simulink model "SGBMDisparity"  (R2021a)
settings: Solver=FixedStepDiscrete  StartTime=0.0  StopTime=simT  FixedStep=1  RelTol=1e-3
PreLoadFcn:
  | DL128 = Simulink.Variant('disparityLevels==128');
  | 
  | DLnot128 = Simulink.Variant('disparityLevels ~= 128');
  | 
  | disparityLevels = 64;
  | 
  | imgRowSize = 480;
  | 
  | imgColSize = 640;
  | 
  | P2 = 200; % Smoothness Penalty Large
  | P1 = 15;  % Smoothness Penalty Small
  | 
  | disparityFactor = 16;
  | 
  | uniquenessRatio = 5;
  | 
  | p = imgColSize - 1;
  | q = imgRowSize * imgColSize -1;
  | r = imgColSize - disparityLevels -1;
  | s = (imgRowSize*(imgColSize-disparityLevels))-1;
  | 
  | simT = 800*525
  | 
  | dtGain = 4;
InitFcn:
  | DL128 = Simulink.Variant('disparityLevels==128');
  | 
  | DLnot128 = Simulink.Variant('disparityLevels ~= 128');
  | 
  | img = imread(get_param('SGBMDisparity/stereoImage','FileName'));
  | 
  | [imgRowSize, imgColSize,chn] = size(img);
  | 
  | P2 = 200; % Smoothness Penalty Large
  | P1 = 15;  % Smoothness Penalty Small
  | 
  | disparityFactor = 16;
  | 
  | uniquenessRatio = str2num(get_param('SGBMDisparity/SGBMHDLAlgorithm/SGBMHDLAlgorithmWorker','UT'));
  | 
  | disparityLevels = str2num(get_param('SGBMDisparity/SGBMHDLAlgorithm/SGBMHDLAlgorithmWorker','DL'));
  | 
  | p = imgColSize - 1;
  | q = imgRowSize * imgColSize -1;
  | r = imgColSize - disparityLevels -1;
  | s = (imgRowSize*(imgColSize-disparityLevels))-1;
  | 
  | if imgRowSize == 720 && imgColSize == 1280
  | simT = 1650*750;
  | elseif imgRowSize == 540 && imgColSize == 960
  | simT = 1050*600;
  | elseif imgRowSize == 480 && imgColSize == 640
  | simT = 800*525;
  | end
  | 
  | %if imgRowSize == 720 && imgColSize == 1280
  | %dtGain = 2;
  | %elseif imgRowSize == 540 && imgColSize == 960
  | %dtGain = 2.6;
  | %elseif imgRowSize == 480 && imgColSize == 640
  | %dtGain = 4;
  | %end
  | 
  | dtGain = 8;
libraries: simulink x331, hdlsllib x113, visionhdlutilities x9, visionhdlio x2, visionsources x1
(part 1 of 6)
settings Model: DataTypeOverride=Off  SimulationMode=accelerator  Creator=The MathWorks, Inc.  LastModifiedBy=user
settings SolverCC: AlgebraicLoopSolver=TrustRegion  AutoInsertRateTranBlk=on
settings DataIOCC: LimitDataPoints=on  SaveOutput=off  SignalLogging=off  SaveTime=off  ReturnWorkspaceOutputs=off
settings OptimizationCC: BlockReduction=off  ConditionallyExecuteInputs=off  DefaultParameterBehavior=Inlined  LifeSpan=inf
settings DebuggingCC: AlgebraicLoopMsg=error  SingleTaskRateTransMsg=error  AllowSymbolicDim=off  StrictBusMsg=ErrorOnBusTreatedAsVector  SFUnexpectedBacktrackingDiag=warning  SFNoUnconditionalDefaultTransitionDiag=warning  SFExecutionAtInitializationDiag=none  SFMachineParentedDataDiag=warning  ArithmeticOperatorsInVariantConditions=warning
settings HardwareCC: ProdBitPerPointer=32  ProdBitPerSizeT=32  ProdBitPerPtrDiffT=32  ProdLargestAtomicFloat=None  ProdIntDivRoundTo=Undefined  ProdEndianess=Unspecified  ProdWordSize=32  ProdHWDeviceType=ASIC/FPGA->ASIC/FPGA  ProdEqTarget=off
settings SFSimCC: SimUseLocalCustomCode=off  CustomCodeUndefinedFunction=UseInterfaceOnly
settings RTWCC: RTWUseLocalCustomCode=off
settings CodeAppCC: StateflowObjectComments=on
settings GRTTargetCC: TargetLangStandard=C89/C90 (ANSI)
settings ConfigComp: CovMetricSettings=dw  CovSaveCumulativeToWorkspaceVar=on  CovSaveSingleToWorkspaceVar=on  CovExternalEMLEnable=off  CovSFcnEnable=off

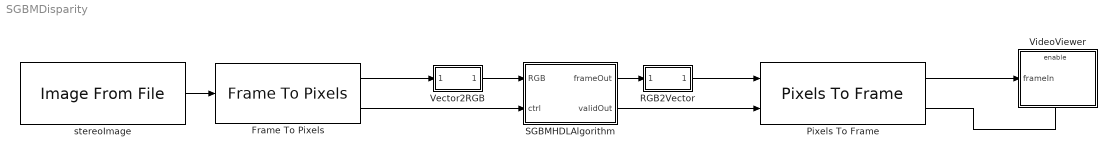
== system SGBMDisparity ==
  Frame To Pixels : visionhdlio/Frame To Pixels  NumComponents=3  NumPixels=1  VideoFormat=480p  ActivePixelsPerLine=imgColSize  ActiveVideoLines=imgRowSize  TotalPixelsPerLine=imgColSize+90  TotalVideoLines=imgRowSize+60  StartingActiveLine=31  FrontPorch=45  SampleTime=0
      settings: SourceProductBaseCode=VT
  Pixels To Frame : visionhdlio/Pixels To Frame  NumComponents=3  NumPixels=1  VideoFormat=480p  ActivePixelsPerLine=imgColSize  ActiveVideoLines=imgRowSize  TotalPixelsPerLine=imgColSize+90  TotalVideoLines=imgRowSize+60
      settings: SourceProductBaseCode=VT
  RGB2Vector : Subsystem
  SGBMHDLAlgorithm : Subsystem  TreatAsAtomicUnit=on
  Vector2RGB : Subsystem
  VideoViewer : Subsystem
  stereoImage : visionsources/Image From File  Tag=vipblks_nd  FileName=D:\Work\XilFPGAdev\Custom_IP_Cores\SimulinkHDLCoder\SGBMDisparity\stereoTestimg_01_480p.bmp  Ts=simT  imagePorts=One multidimensional signal  OutPortLabels=R|G|B  ImageDataType=Inherit from input image  sdImageDataType=uint(8)  Signed=on  WordLength=16  FractionLengthMode=User-defined  FractionLength=15
  wires:
  stereoImage/1 -> Frame To Pixels/1
  Pixels To Frame/1 -> VideoViewer/1(frameIn)
  Pixels To Frame/2 -> VideoViewer/Enable
  Frame To Pixels/1 -> Vector2RGB/1(RGBVector)
  Frame To Pixels/2 -> SGBMHDLAlgorithm/2(ctrl)
  SGBMHDLAlgorithm/1(frameOut) -> RGB2Vector/1(RGB)
  SGBMHDLAlgorithm/2(validOut) -> Pixels To Frame/2
  Vector2RGB/1(RGB) -> SGBMHDLAlgorithm/1(RGB)
  RGB2Vector/1(RGBVector) -> Pixels To Frame/1

== system SGBMDisparity/RGB2Vector ==
  note: RGB represented in
      | 32'hFFRRGGBB
  RGB : Inport
  Bit Slice : hdlsllib/Logic and Bit Operations/Bit Slice  lidx=23  ridx=16
      settings: SourceProductBaseCode=SL
  Bit Slice1 : hdlsllib/Logic and Bit Operations/Bit Slice  lidx=15  ridx=8
      settings: SourceProductBaseCode=SL
  Bit Slice2 : hdlsllib/Logic and Bit Operations/Bit Slice  lidx=7  ridx=0
      settings: SourceProductBaseCode=SL
  Mux : Mux  Inputs=3
  Signal Specification : SignalSpecification
  Transpose : Math  Operator=transpose  SignedPower=on  SaturateOnIntegerOverflow=on
  RGBVector : Outport  VectorParamsAs1DForOutWhenUnconnected=off
  wires:
  Mux/1 -> Transpose/1
  Bit Slice/1 -> Mux/1
  Bit Slice2/1 -> Mux/3
  Bit Slice1/1 -> Mux/2
  RGB/1 -> Bit Slice2/1, Bit Slice1/1, Bit Slice/1
  Transpose/1 -> Signal Specification/1
  Signal Specification/1 -> RGBVector/1

== system SGBMDisparity/SGBMHDLAlgorithm ==
  RGB : Inport
  ctrl : Inport  Port=2
  Bit Concat : hdlsllib/Logic and Bit Operations/Bit Concat  numInputs=4
  Demux : Demux  Outputs=3
  FF : Constant  Value=255  OutDataTypeStr=uint8  SampleTime=-1
  Output : Subsystem
  RGB2Vector : Subsystem
  SGBMHDLAlgorithmWorker : Subsystem  mask{DL=16, UT=5}
      mask prompts: DL "Disparity Levels"; UT "Uniqueness Threshold"
      mask DialogControl Container3 Prompt: Select Disparity Levels
      mask DialogControl Container6 Prompt: Select Uniqueness Threshold
  frameOut : Outport
  validOut : Outport  Port=2
  wires:
  Output/2(validOut) -> validOut/1
  Demux/2 -> SGBMHDLAlgorithmWorker/2(pixelRight)
  SGBMHDLAlgorithmWorker/2(ctrlDisparity) -> Output/2(busIn)
  Demux/1 -> SGBMHDLAlgorithmWorker/1(pixelLeft)
  SGBMHDLAlgorithmWorker/1(pixelDisparity) -> Output/1(pixelIn)
  ctrl/1 -> SGBMHDLAlgorithmWorker/3(ctrl)
  RGB/1 -> RGB2Vector/1(RGB)
  RGB2Vector/1(RGBVector) -> Demux/1
  Bit Concat/1 -> frameOut/1
  FF/1 -> Bit Concat/1
  Output/1(frameOut) -> Bit Concat/4, Bit Concat/2, Bit Concat/3

== system SGBMDisparity/Vector2RGB ==
  note: Encode RGB into 32 bit representation
      | 32'hFFRRGGBB
  RGBVector : Inport
  Bit Concat : hdlsllib/Logic and Bit Operations/Bit Concat  numInputs=4
  Demux : Demux  Outputs=3
  FF : Constant  Value=255  OutDataTypeStr=uint8  SampleTime=-1
  RGB : Outport  VectorParamsAs1DForOutWhenUnconnected=off
  wires:
  Bit Concat/1 -> RGB/1
  RGBVector/1 -> Demux/1
  FF/1 -> Bit Concat/1
  Demux/1 -> Bit Concat/2
  Demux/2 -> Bit Concat/3
  Demux/3 -> Bit Concat/4

== system SGBMDisparity/VideoViewer ==
  frameIn : Inport
  Enable : EnablePort
  HDL Video Viewer : VideoViewer  useColorMap=on  FigPos=[348 749 756 478]
  wires:
  frameIn/1 -> HDL Video Viewer/1

== system SGBMDisparity/SGBMHDLAlgorithm/Output ==
  pixelIn : Inport
  busIn : Inport  Port=2
  Bus Selector : BusSelector  OutputSignals=valid,vStart
  Compare To Constant : simulink/Logic and Bit Operations/Compare To Constant  relop=<=  const=imgColSize-1  OutDataTypeStr=boolean
  Compare To Constant1 : simulink/Logic and Bit Operations/Compare To Constant  relop=<=  const=disparityLevels-1  OutDataTypeStr=boolean
  Constant : Constant  Value=0  OutDataTypeStr=boolean  SampleTime=-1
  Constant1 : Constant  OutDataTypeStr=boolean  SampleTime=-1
  Constant2 : Constant  Value=0  OutDataTypeStr=fixdt(1,14,5)  SampleTime=-1
  Data Type Conversion : DataTypeConversion  OutDataTypeStr=uint8
  Gain : Gain  Gain=dtGain
  HDL Counter : hdlsllib/Sources/HDL Counter  CountType=Count limited  CountInit=0  CountStep=1  CountMax=imgColSize-1  CountFromType=Initial value  CountFrom=0  CountResetPort=off  CountLoadPort=off  CountEnbPort=on  CountDirPort=off  CountHitOutputPort=off  CountDataType=Unsigned  CountWordLen=ceil(log2(imgColSize-1))  CountFracLen=0  CountSampTime=1
  Logical Operator : Logic  AllPortsSameDT=off  OutDataTypeStr=boolean
  Logical Operator1 : Logic  Operator=OR  AllPortsSameDT=off  OutDataTypeStr=boolean
  Logical Operator2 : Logic  Operator=OR  AllPortsSameDT=off  OutDataTypeStr=boolean
  Switch : Switch  Criteria=u2 ~= 0
  Switch1 : Switch  Criteria=u2 ~= 0
  Terminator : Terminator
  To Workspace : ToWorkspace  VariableName=dispMap  SampleTime=-1
      settings: Save2DSignal=2-D array (concatenate along first dimension)
  To Workspace1 : ToWorkspace  VariableName=dispMapValid  SampleTime=-1
      settings: Save2DSignal=2-D array (concatenate along first dimension)
  pixelBusGenerator : Subsystem  mask{hEnd=p, vEnd=q}
      mask prompts: hEnd "hEnd Count"; vEnd "vEnd Count"
      mask DialogControl DescGroupVar Prompt: Counter Values
  frameOut : Outport  VectorParamsAs1DForOutWhenUnconnected=off
  validOut : Outport  Port=2  VectorParamsAs1DForOutWhenUnconnected=off
  wires:
  pixelBusGenerator/1(busOut) -> validOut/1
  Switch1/1 -> Gain/1, To Workspace/1
  busIn/1 -> Bus Selector/1
  Gain/1 -> Data Type Conversion/1
  Data Type Conversion/1 -> frameOut/1
  Constant/1 -> Switch/3
  Constant1/1 -> Switch/1
  HDL Counter/1 -> Compare To Constant/1, Compare To Constant1/1
  Compare To Constant/1 -> Logical Operator/2
  Logical Operator1/1 -> HDL Counter/1
  Compare To Constant1/1 -> Logical Operator2/2, Logical Operator1/2
  Bus Selector/1 -> Switch1/2, Logical Operator/1, Logical Operator1/1  "<valid>"
  Logical Operator/1 -> Logical Operator2/1
  Logical Operator2/1 -> Switch/2
  Constant2/1 -> Switch1/3
  pixelIn/1 -> Switch1/1
  Switch/1 -> To Workspace1/1, pixelBusGenerator/1(validIn)
  Bus Selector/2 -> Terminator/1  "<vStart>"

== system SGBMDisparity/SGBMHDLAlgorithm/RGB2Vector ==
  note: RGB represented in
      | 32'hFFRRGGBB
  RGB : Inport
  Bit Slice : hdlsllib/Logic and Bit Operations/Bit Slice  lidx=23  ridx=16
      settings: SourceProductBaseCode=SL
  Bit Slice1 : hdlsllib/Logic and Bit Operations/Bit Slice  lidx=15  ridx=8
      settings: SourceProductBaseCode=SL
  Bit Slice2 : hdlsllib/Logic and Bit Operations/Bit Slice  lidx=7  ridx=0
      settings: SourceProductBaseCode=SL
  Mux : Mux  Inputs=3
  RGBVector : Outport  VectorParamsAs1DForOutWhenUnconnected=off
  wires:
  Bit Slice/1 -> Mux/1
  Bit Slice2/1 -> Mux/3
  Bit Slice1/1 -> Mux/2
  RGB/1 -> Bit Slice2/1, Bit Slice1/1, Bit Slice/1
  Mux/1 -> RGBVector/1

== system SGBMDisparity/SGBMHDLAlgorithm/SGBMHDLAlgorithmWorker ==
  pixelLeft : Inport
  pixelRight : Inport  Port=2
  ctrl : Inport  Port=3
  DirectionalCost : Subsystem
  MatchingCost : Subsystem
  PostProcessing : Subsystem
  pixelDisparity : Outport  VectorParamsAs1DForOutWhenUnconnected=off
  ctrlDisparity : Outport  Port=2  VectorParamsAs1DForOutWhenUnconnected=off
  wires:
  PostProcessing/1(disparityOut) -> pixelDisparity/1
  PostProcessing/2(busOut) -> ctrlDisparity/1
  pixelLeft/1 -> MatchingCost/1(pixelLeft)
  pixelRight/1 -> MatchingCost/2(pixelRight)
  ctrl/1 -> MatchingCost/3(busIn)
  MatchingCost/1(hammDistA) -> DirectionalCost/1(matchCostA)
  MatchingCost/2(hammDistValidA) -> DirectionalCost/2(busA)
  MatchingCost/3(hammDistRL) -> DirectionalCost/3(matchCostRL)
  MatchingCost/4(hammDistValidRL) -> DirectionalCost/4(busRL)
  DirectionalCost/2(validOut) -> PostProcessing/2(validIn)
  DirectionalCost/1(totalCostOut) -> PostProcessing/1(totalCostIn)

== system SGBMDisparity/SGBMHDLAlgorithm/Output/pixelBusGenerator ==
  validIn : Inport
  Horizontal : hdlsllib/Sources/HDL Counter  CountType=Count limited  CountInit=0  CountStep=1  CountMax=hEnd  CountFromType=Initial value  CountFrom=0  CountResetPort=off  CountLoadPort=off  CountEnbPort=on  CountDirPort=off  CountHitOutputPort=off  CountDataType=Unsigned  CountWordLen=ceil(log2(hEnd))  CountFracLen=0  CountSampTime=1
  Logical Operator{3..6} (4 alike) : Logic  AllPortsSameDT=off  OutDataTypeStr=boolean
  Pixel Control Bus Creator : visionhdlutilities/Pixel Control Bus Creator
      settings: SourceProductBaseCode=VT
  Vertical : hdlsllib/Sources/HDL Counter  CountType=Count limited  CountInit=0  CountStep=1  CountMax=vEnd  CountFromType=Initial value  CountFrom=0  CountResetPort=off  CountLoadPort=off  CountEnbPort=on  CountDirPort=off  CountHitOutputPort=off  CountDataType=Unsigned  CountWordLen=ceil(log2(vEnd))  CountFracLen=0  CountSampTime=1
  hEnd : simulink/Logic and Bit Operations/Compare To Constant  relop===  const=hEnd  OutDataTypeStr=boolean
  hStart : simulink/Logic and Bit Operations/Compare To Constant  relop===  const=0  OutDataTypeStr=boolean
  vEnd : simulink/Logic and Bit Operations/Compare To Constant  relop===  const=vEnd  OutDataTypeStr=boolean
  vStart : simulink/Logic and Bit Operations/Compare To Constant  relop===  const=0  OutDataTypeStr=boolean
  busOut : Outport  VectorParamsAs1DForOutWhenUnconnected=off
  wires:
  validIn/1 -> Pixel Control Bus Creator/5, Vertical/1, Logical Operator4/1, Logical Operator5/1, Logical Operator6/1, Logical Operator3/1, Horizontal/1
  Horizontal/1 -> hEnd/1, hStart/1
  hEnd/1 -> Logical Operator4/2
  Vertical/1 -> vStart/1, vEnd/1
  vStart/1 -> Logical Operator5/2
  vEnd/1 -> Logical Operator6/2
  Logical Operator5/1 -> Pixel Control Bus Creator/3
  Logical Operator3/1 -> Pixel Control Bus Creator/1
  Logical Operator4/1 -> Pixel Control Bus Creator/2
  hStart/1 -> Logical Operator3/2
  Logical Operator6/1 -> Pixel Control Bus Creator/4
  Pixel Control Bus Creator/1 -> busOut/1

== system SGBMDisparity/SGBMHDLAlgorithm/SGBMHDLAlgorithmWorker/DirectionalCost ==
  matchCostA : Inport
  busA : Inport  Port=2
  matchCostRL : Inport  Port=3
  busRL : Inport  Port=4
  Bus Selector{,1..4} (5 alike) : BusSelector  OutputSignals=valid
  Delay{,1..4,6,16..17} (8 alike) : Delay  DelayLength=6
  Delay{5,7..11,14..15,18..19} (10 alike) : Delay  DelayLength=1
  Delay12 : Delay
  Delay13 : Delay
  LeftToRight : Subsystem
  Logical Operator{,1..3} (4 alike) : Logic  AllPortsSameDT=off  OutDataTypeStr=boolean
  RightToLeft : Subsystem
  Sum : Sum  Inputs=|++
  Sum1 : Sum  Inputs=|++
  Sum2 : Sum  Inputs=|++
  Sum3 : Sum  Inputs=|++  OutDataTypeStr=fixdt(1,13,0)
  TopLeftToBottomRight : Subsystem
  TopRightToBottomLeft : Subsystem
  TopToBottom : Subsystem
  totalCostOut : Outport  VectorParamsAs1DForOutWhenUnconnected=off
  validOut : Outport  Port=2  VectorParamsAs1DForOutWhenUnconnected=off
  wires:
  busA/1 -> TopRightToBottomLeft/2(busIn), TopToBottom/2(busIn), TopLeftToBottomRight/2(busIn), LeftToRight/2(busIn)
  matchCostRL/1 -> RightToLeft/1(matchCostIn)
  busRL/1 -> RightToLeft/2(busIn)
  matchCostA/1 -> TopRightToBottomLeft/1(matchCostIn), TopToBottom/1(matchCostIn), TopLeftToBottomRight/1(matchCostIn), LeftToRight/1(matchCostIn)
  Bus Selector3/1 -> Logical Operator1/2  "<valid>"
  Delay12/1 -> Sum3/2
  Logical Operator/1 -> Delay11/1
  Sum3/1 -> Delay8/1
  Bus Selector2/1 -> Logical Operator/2  "<valid>"
  Logical Operator1/1 -> Delay7/1
  Delay15/1 -> Bus Selector4/1
  Delay1/1 -> Sum1/1
  Delay14/1 -> Delay12/1
  Delay18/1 -> Sum3/1
  Delay10/1 -> Sum2/1
  Logical Operator3/1 -> Delay9/1
  Delay17/1 -> Bus Selector3/1
  Delay11/1 -> Logical Operator2/1
  TopRightToBottomLeft/1(trblOut) -> Delay16/1
  Logical Operator2/1 -> Delay19/1
  Delay19/1 -> Logical Operator3/1
  TopToBottom/2(tbBus) -> Delay3/1
  TopToBottom/1(tbOut) -> Delay1/1
  Bus Selector1/1 -> Logical Operator1/1  "<valid>"
  Bus Selector4/1 -> Delay13/1  "<valid>"
  Sum1/1 -> Delay5/1
  Delay6/1 -> Bus Selector2/1
  Delay7/1 -> Logical Operator2/2
  TopRightToBottomLeft/2(trblBus) -> Delay17/1
  RightToLeft/1(rlCost) -> Delay14/1
  TopLeftToBottomRight/1(tlbrCost) -> Delay4/1
  RightToLeft/2(rlBus) -> Delay15/1
  Delay3/1 -> Bus Selector1/1
  Bus Selector/1 -> Logical Operator/1  "<valid>"
  Delay4/1 -> Sum/2
  Delay/1 -> Sum/1
  Delay2/1 -> Bus Selector/1
  Delay9/1 -> validOut/1
  Sum/1 -> Delay10/1
  TopLeftToBottomRight/2(tlbrBus) -> Delay6/1
  Delay13/1 -> Logical Operator3/2
  LeftToRight/2(lrBus) -> Delay2/1
  Sum2/1 -> Delay18/1
  LeftToRight/1(lrCost) -> Delay/1
  Delay5/1 -> Sum2/2
  Delay16/1 -> Sum1/2
  Delay8/1 -> totalCostOut/1

== system SGBMDisparity/SGBMHDLAlgorithm/SGBMHDLAlgorithmWorker/MatchingCost ==
  pixelLeft : Inport
  pixelRight : Inport  Port=2
  busIn : Inport  Port=3
  Bus Selector : BusSelector  OutputSignals=valid
  Bus Selector1 : BusSelector  OutputSignals=valid
  CensusTransform : Subsystem
  CensusTransform1 : Subsystem
  HammDistA : Subsystem
  HammDistRL : Subsystem
  To Workspace1 : ToWorkspace  Commented=on  VariableName=Hamm_sim_RL  SampleTime=-1
      settings: Save2DSignal=2-D array (concatenate along first dimension)
  To Workspace2 : ToWorkspace  Commented=on  VariableName=Hamm_Valid_RL  SampleTime=-1
      settings: Save2DSignal=2-D array (concatenate along first dimension)
  To Workspace4 : ToWorkspace  Commented=on  VariableName=Hamm_sim_A  SampleTime=-1
      settings: Save2DSignal=2-D array (concatenate along first dimension)
  To Workspace5 : ToWorkspace  Commented=on  VariableName=Hamm_Valid_A  SampleTime=-1
      settings: Save2DSignal=2-D array (concatenate along first dimension)
  hammDistA : Outport  VectorParamsAs1DForOutWhenUnconnected=off
  hammDistValidA : Outport  Port=2  VectorParamsAs1DForOutWhenUnconnected=off
  hammDistRL : Outport  Port=3  VectorParamsAs1DForOutWhenUnconnected=off
  hammDistValidRL : Outport  Port=4  VectorParamsAs1DForOutWhenUnconnected=off
  wires:
  HammDistRL/1(hammDist) -> To Workspace1/1, hammDistRL/1
  HammDistRL/2(busOut) -> Bus Selector1/1, hammDistValidRL/1
  HammDistA/2(busOut) -> Bus Selector/1, hammDistValidA/1
  pixelLeft/1 -> CensusTransform/1(pixelIn)
  pixelRight/1 -> CensusTransform1/1(pixelIn)
  busIn/1 -> CensusTransform1/2(ctrlIn), CensusTransform/2(ctrlIn)
  CensusTransform1/2(busRight) -> HammDistA/4(rightBus), HammDistRL/4(rightBus)
  CensusTransform/2(busLeft) -> HammDistRL/2(leftBus), HammDistA/2(leftBus)
  CensusTransform/1(ctLeft) -> HammDistRL/1(leftIn), HammDistA/1(leftIn)
  CensusTransform1/1(ctRight) -> HammDistA/3(rightIn), HammDistRL/3(rightIn)
  HammDistA/1(hammDist) -> To Workspace4/1, hammDistA/1
  Bus Selector/1 -> To Workspace5/1  "<valid>"
  Bus Selector1/1 -> To Workspace2/1  "<valid>"

== system SGBMDisparity/SGBMHDLAlgorithm/SGBMHDLAlgorithmWorker/PostProcessing ==
  totalCostIn : Inport
  validIn : Inport  Port=2
  Constant : Constant  Value=0  OutDataTypeStr=fixdt(1,14,5)  SampleTime=-1
  Constant1 : Constant  Value=0  OutDataTypeStr=uint8  SampleTime=-1
  Constant2 : Constant  Value=-1  OutDataTypeStr=fixdt(1,14,5)  SampleTime=-1
  Data Type Conversion : DataTypeConversion  OutDataTypeStr=fixdt(1,14,5)
  Delay : Delay  DelayLength=7
  Delay1 : Delay  DelayLength=22
  Delay{3..7,14} (6 alike) : Delay  DelayLength=1
  Delay2 : Delay  DelayLength=22
  Interpolation : Subsystem
  Logical Operator1 : Logic  AllPortsSameDT=off  OutDataTypeStr=boolean
  Relational Operator : RelationalOperator  Operator=<  OutDataTypeStr=boolean  RndMeth=Nearest
  Switch : Switch  Criteria=u2 ~= 0
  Switch1 : Switch  Criteria=u2 ~= 0
  UniquenessFcn : Subsystem
  pixelBusGenerator : Subsystem  mask{hEnd=r, vEnd=s}
      mask prompts: hEnd "hEnd Count"; vEnd "vEnd Count"
      mask DialogControl DescGroupVar Prompt: Counter Values
  disparityOut : Outport  VectorParamsAs1DForOutWhenUnconnected=off
  busOut : Outport  Port=2  VectorParamsAs1DForOutWhenUnconnected=off
  wires:
  totalCostIn/1 -> Delay/1, Interpolation/1(totalCostIn)
  Interpolation/3(validOutUNF) -> UniquenessFcn/4(validIn)
  Interpolation/2(minIndex) -> UniquenessFcn/3(minIndex)
  Interpolation/1(minIndexVal) -> UniquenessFcn/2(minIndexVal)
  Delay/1 -> UniquenessFcn/1(totalCostIn)
  Delay1/1 -> Logical Operator1/1
  UniquenessFcn/2(validOut) -> Delay1/1
  UniquenessFcn/1(UNF) -> Delay2/1
  Delay2/1 -> Switch/2
  Constant/1 -> Switch/1
  Interpolation/4(disparity) -> Data Type Conversion/1
  Constant1/1 -> Relational Operator/2
  Constant2/1 -> Switch1/1
  Delay3/1 -> Relational Operator/1, Switch1/3
  Relational Operator/1 -> Switch1/2
  Switch/1 -> Delay3/1
  Logical Operator1/1 -> Delay4/1
  Delay4/1 -> Delay5/1
  Switch1/1 -> Delay6/1
  Delay6/1 -> disparityOut/1
  Delay14/1 -> Switch/3
  Delay7/1 -> Logical Operator1/2
  pixelBusGenerator/1(busOut) -> busOut/1
  Interpolation/5(validOut) -> Delay7/1
  Delay5/1 -> pixelBusGenerator/1(validIn)
  Data Type Conversion/1 -> Delay14/1
  validIn/1 -> Interpolation/2(validIn)

== system SGBMDisparity/SGBMHDLAlgorithm/SGBMHDLAlgorithmWorker/DirectionalCost/LeftToRight ==
  matchCostIn : Inport
  busIn : Inport  Port=2
  Bus Selector : BusSelector  OutputSignals=vStart,valid
  Compare To Constant : simulink/Logic and Bit Operations/Compare To Constant  relop=<  const=imgColSize-disparityLevels-1  OutDataTypeStr=boolean
  Delay1 : Delay  DelayLength=1
  Delay2 : Delay  DelayLength=1
  Delay3 : Delay  DelayLength=1
  HDL Counter : hdlsllib/Sources/HDL Counter  CountType=Count limited  CountInit=0  CountStep=1  CountMax=imgColSize-disparityLevels-1  CountFromType=Initial value  CountFrom=0  CountResetPort=on  CountLoadPort=off  CountEnbPort=on  CountDirPort=off  CountHitOutputPort=off  CountDataType=Unsigned  CountWordLen=ceil(log2(imgColSize-disparityLevels-1))  CountFracLen=0  CountSampTime=1
  lrSubsystem : Subsystem
  lrCost : Outport  VectorParamsAs1DForOutWhenUnconnected=off
  lrBus : Outport  Port=2  VectorParamsAs1DForOutWhenUnconnected=off
  wires:
  Bus Selector/2 -> Delay3/1  "<valid>"
  Bus Selector/1 -> HDL Counter/1  "<vStart>"
  busIn/1 -> Delay1/1, Bus Selector/1
  matchCostIn/1 -> Delay2/1
  Delay1/1 -> lrBus/1
  lrSubsystem/1(lrCost) -> lrCost/1
  HDL Counter/1 -> Compare To Constant/1
  Compare To Constant/1 -> lrSubsystem/1(enable)
  Delay2/1 -> lrSubsystem/2(matchCostIn)
  Delay3/1 -> lrSubsystem/Enable, HDL Counter/2

== system SGBMDisparity/SGBMHDLAlgorithm/SGBMHDLAlgorithmWorker/DirectionalCost/RightToLeft ==
  matchCostIn : Inport
  busIn : Inport  Port=2
  Bus Selector1 : BusSelector  OutputSignals=vStart,valid
  Compare To Constant : simulink/Logic and Bit Operations/Compare To Constant  relop=<  const=imgColSize-disparityLevels-1  OutDataTypeStr=boolean
  Delay{1..4,6} (5 alike) : Delay  DelayLength=1
  HDL Counter : hdlsllib/Sources/HDL Counter  CountType=Count limited  CountInit=0  CountStep=1  CountMax=imgColSize-disparityLevels-1  CountFromType=Initial value  CountFrom=0  CountResetPort=on  CountLoadPort=off  CountEnbPort=on  CountDirPort=off  CountHitOutputPort=off  CountDataType=Unsigned  CountWordLen=ceil(log2(imgColSize-disparityLevels-1))  CountFracLen=0  CountSampTime=1
  InverseRow_ForEach : Subsystem  TreatAsAtomicUnit=on
  Logical Operator : Logic  Inputs=1  AllPortsSameDT=off  OutDataTypeStr=boolean
  pixelBusGenerator : Subsystem  mask{hEnd=r, vEnd=s}
      mask prompts: hEnd "hEnd Count"; vEnd "vEnd Count"
      mask DialogControl DescGroupVar Prompt: Counter Values
  rlSubsystem : Subsystem
  rlCost : Outport  VectorParamsAs1DForOutWhenUnconnected=off
  rlBus : Outport  Port=2  VectorParamsAs1DForOutWhenUnconnected=off
  wires:
  Bus Selector1/2 -> Delay2/1  "<valid>"
  pixelBusGenerator/1(busOut) -> rlBus/1
  InverseRow_ForEach/1(Out) -> rlCost/1
  InverseRow_ForEach/2(valid_Out) -> Logical Operator/1
  Logical Operator/1 -> pixelBusGenerator/1(validIn)
  matchCostIn/1 -> Delay3/1
  Bus Selector1/1 -> HDL Counter/1  "<vStart>"
  busIn/1 -> Delay4/1, Bus Selector1/1
  rlSubsystem/1(Out1) -> Delay6/1
  Delay6/1 -> InverseRow_ForEach/1(In)
  Delay1/1 -> InverseRow_ForEach/2(busIn)
  HDL Counter/1 -> Compare To Constant/1
  Compare To Constant/1 -> rlSubsystem/1(enable)
  Delay2/1 -> HDL Counter/2, rlSubsystem/Enable
  Delay3/1 -> rlSubsystem/2(matchCostIn)
  Delay4/1 -> Delay1/1

== system SGBMDisparity/SGBMHDLAlgorithm/SGBMHDLAlgorithmWorker/DirectionalCost/TopLeftToBottomRight ==
  matchCostIn : Inport
  busIn : Inport  Port=2
  Bus Selector : BusSelector  OutputSignals=vStart,valid
  CC : simulink/Logic and Bit Operations/Compare To Constant  relop=<  const=imgColSize-disparityLevels-1  OutDataTypeStr=boolean
  Delay : Delay  DelayLength=1
  Delay1 : Delay  DelayLength=1
  Delay2 : Delay  DelayLength=1
  HDL Counter : hdlsllib/Sources/HDL Counter  CountType=Count limited  CountInit=0  CountStep=1  CountMax=imgColSize-disparityLevels-1  CountFromType=Initial value  CountFrom=0  CountResetPort=on  CountLoadPort=off  CountEnbPort=on  CountDirPort=off  CountHitOutputPort=off  CountDataType=Unsigned  CountWordLen=ceil(log2(imgColSize-disparityLevels-1))  CountFracLen=0  CountSampTime=1
  LO : Logic  IconShape=distinctive  AllPortsSameDT=off  OutDataTypeStr=boolean
  tlbrSubsystem : Subsystem
  tlbrCost : Outport  VectorParamsAs1DForOutWhenUnconnected=off
  tlbrBus : Outport  Port=2  VectorParamsAs1DForOutWhenUnconnected=off
  wires:
  busIn/1 -> Delay2/1, Bus Selector/1
  Bus Selector/1 -> HDL Counter/1  "<vStart>"
  Bus Selector/2 -> Delay/1  "<valid>"
  matchCostIn/1 -> Delay1/1
  CC/1 -> LO/2
  HDL Counter/1 -> CC/1
  LO/1 -> tlbrSubsystem/1(enable)
  Delay/1 -> HDL Counter/2, tlbrSubsystem/Enable, LO/1
  tlbrSubsystem/1(tlbrCost) -> tlbrCost/1
  Delay2/1 -> tlbrBus/1
  Delay1/1 -> tlbrSubsystem/2(matchCostIn)

== system SGBMDisparity/SGBMHDLAlgorithm/SGBMHDLAlgorithmWorker/DirectionalCost/TopRightToBottomLeft ==
  matchCostIn : Inport
  busIn : Inport  Port=2
  Bus Selector : BusSelector  OutputSignals=vStart,valid
  Compare To Constant : simulink/Logic and Bit Operations/Compare To Constant  relop=>  const=0  OutDataTypeStr=boolean
  Delay : Delay  DelayLength=1
  Delay1 : Delay  DelayLength=1
  Delay2 : Delay  DelayLength=1
  HDL Counter : hdlsllib/Sources/HDL Counter  CountType=Count limited  CountInit=0  CountStep=1  CountMax=imgColSize-disparityLevels-1  CountFromType=Initial value  CountFrom=0  CountResetPort=on  CountLoadPort=off  CountEnbPort=on  CountDirPort=off  CountHitOutputPort=off  CountDataType=Unsigned  CountWordLen=ceil(log2(imgColSize-disparityLevels-1))  CountFracLen=0  CountSampTime=1
  Logical Operator2 : Logic  IconShape=distinctive  AllPortsSameDT=off  OutDataTypeStr=boolean
  trblSubsystem : Subsystem
  trblOut : Outport  VectorParamsAs1DForOutWhenUnconnected=off
  trblBus : Outport  Port=2  VectorParamsAs1DForOutWhenUnconnected=off
  wires:
  busIn/1 -> Delay1/1, Bus Selector/1
  Bus Selector/1 -> HDL Counter/1  "<vStart>"
  Bus Selector/2 -> Delay/1  "<valid>"
  matchCostIn/1 -> Delay2/1
  HDL Counter/1 -> Compare To Constant/1
  Compare To Constant/1 -> Logical Operator2/2
  Logical Operator2/1 -> trblSubsystem/1(enable)
  Delay/1 -> trblSubsystem/Enable, Logical Operator2/1, HDL Counter/2
  Delay1/1 -> trblBus/1
  trblSubsystem/1(trblCost) -> trblOut/1
  Delay2/1 -> trblSubsystem/2(matchCostIn)

== system SGBMDisparity/SGBMHDLAlgorithm/SGBMHDLAlgorithmWorker/DirectionalCost/TopToBottom ==
  matchCostIn : Inport
  busIn : Inport  Port=2
  Bus Selector : BusSelector  OutputSignals=valid
  Delay : Delay  DelayLength=1
  Delay1 : Delay  DelayLength=1
  tbSubsystem : Subsystem
  tbOut : Outport  VectorParamsAs1DForOutWhenUnconnected=off
  tbBus : Outport  Port=2  VectorParamsAs1DForOutWhenUnconnected=off
  wires:
  busIn/1 -> Delay/1, Bus Selector/1
  Bus Selector/1 -> tbSubsystem/1(enable), tbSubsystem/Enable  "<valid>"
  matchCostIn/1 -> tbSubsystem/2(matchCostIn)
  tbSubsystem/1(tbCost) -> Delay1/1
  Delay/1 -> tbBus/1
  Delay1/1 -> tbOut/1

== system SGBMDisparity/SGBMHDLAlgorithm/SGBMHDLAlgorithmWorker/MatchingCost/CensusTransform ==
  pixelIn : Inport
  ctrlIn : Inport  Port=2
  ctLogic : Subsystem
  dataAligner : Subsystem
  validLogic : Subsystem
  zeroPadding : Subsystem
  ctLeft : Outport  VectorParamsAs1DForOutWhenUnconnected=off
  busLeft : Outport  Port=2  VectorParamsAs1DForOutWhenUnconnected=off
  wires:
  pixelIn/1 -> zeroPadding/1(pixelIn)
  ctrlIn/1 -> zeroPadding/2(ctrlIn)
  zeroPadding/1(pixelOut) -> ctLogic/1(pixelIn)
  zeroPadding/2(validOut) -> ctLogic/Enable, validLogic/1(validIn)
  zeroPadding/3(resetOut) -> validLogic/2(reset)
  validLogic/1(busOut) -> dataAligner/2(busIn)
  ctLogic/1(resultOut) -> dataAligner/1(dataIn)
  dataAligner/2(busOut) -> busLeft/1
  dataAligner/1(dataOut) -> ctLeft/1

== system SGBMDisparity/SGBMHDLAlgorithm/SGBMHDLAlgorithmWorker/MatchingCost/CensusTransform1 ==
  pixelIn : Inport
  ctrlIn : Inport  Port=2
  ctLogic : Subsystem
  dataAligner : Subsystem
  validLogic : Subsystem
  zeroPadding : Subsystem
  ctRight : Outport  VectorParamsAs1DForOutWhenUnconnected=off
  busRight : Outport  Port=2  VectorParamsAs1DForOutWhenUnconnected=off
  wires:
  pixelIn/1 -> zeroPadding/1(pixelIn)
  ctrlIn/1 -> zeroPadding/2(ctrlIn)
  zeroPadding/1(pixelOut) -> ctLogic/1(pixelIn)
  zeroPadding/2(validOut) -> ctLogic/Enable, validLogic/1(validIn)
  zeroPadding/3(resetOut) -> validLogic/2(reset)
  ctLogic/1(resultOut) -> dataAligner/1(dataIn)
  validLogic/1(busOut) -> dataAligner/2(busIn)
  dataAligner/1(dataOut) -> ctRight/1
  dataAligner/2(busOut) -> busRight/1

== system SGBMDisparity/SGBMHDLAlgorithm/SGBMHDLAlgorithmWorker/MatchingCost/HammDistA ==
  leftIn : Inport
  leftBus : Inport  Port=2
  rightIn : Inport  Port=3
  rightBus : Inport  Port=4
  Bus Selector : BusSelector  OutputSignals=vStart,valid
  Bus Selector1 : BusSelector  OutputSignals=vStart,valid
  Compare To Constant : simulink/Logic and Bit Operations/Compare To Constant  relop=>=  const=disparityLevels  OutDataTypeStr=boolean
  Constant : Constant  Value=0  OutDataTypeStr=boolean  SampleTime=-1
  Constant1 : Constant  OutDataTypeStr=boolean  SampleTime=-1
  Delay{,3..5} (4 alike) : Delay  DelayLength=1
  Delay{1..2,6..7,64,66} (6 alike) : Delay  DelayLength=2*imgColSize - disparityLevels
  Delay31 : Delay  DelayLength=5
  HDL Counter : hdlsllib/Sources/HDL Counter  CountType=Count limited  CountInit=0  CountStep=1  CountMax=imgColSize-1  CountFromType=Initial value  CountFrom=0  CountResetPort=on  CountLoadPort=off  CountEnbPort=on  CountDirPort=off  CountHitOutputPort=off  CountDataType=Unsigned  CountWordLen=ceil(log2(imgColSize))  CountFracLen=0  CountSampTime=1
  Int2Bin : Subsystem
  Logical Operator : Logic  AllPortsSameDT=off  OutDataTypeStr=boolean
  Logical Operator1 : Logic  AllPortsSameDT=off  OutDataTypeStr=boolean
  Logical Operator2 : Logic  AllPortsSameDT=off  OutDataTypeStr=boolean
  Switch : Switch  Criteria=u2 ~= 0
  enabledTappedDelay : Subsystem
  hammDispForEach : Subsystem  TreatAsAtomicUnit=on
  pixelBusGenerator : Subsystem  mask{hEnd=r, vEnd=s}
      mask prompts: hEnd "hEnd Count"; vEnd "vEnd Count"
      mask DialogControl DescGroupVar Prompt: Counter Values
  hammDist : Outport  VectorParamsAs1DForOutWhenUnconnected=off
  busOut : Outport  Port=2  VectorParamsAs1DForOutWhenUnconnected=off
  wires:
  rightIn/1 -> Delay66/1
  leftIn/1 -> Delay64/1
  Bus Selector/2 -> Delay7/1  "<valid>"
  Logical Operator/1 -> Logical Operator1/2, HDL Counter/2
  Constant/1 -> Switch/3
  Bus Selector1/2 -> Delay2/1  "<valid>"
  Constant1/1 -> Switch/1
  HDL Counter/1 -> Compare To Constant/1
  Switch/1 -> Delay31/1
  pixelBusGenerator/1(busOut) -> busOut/1
  hammDispForEach/1(hammDist) -> hammDist/1
  Delay64/1 -> Delay4/1
  Int2Bin/1(binOut) -> hammDispForEach/1(leftCSCTIn)
  Delay66/1 -> Delay5/1
  enabledTappedDelay/1(pixelOut) -> hammDispForEach/2(rightCSCTIn)
  Compare To Constant/1 -> Logical Operator1/1
  Logical Operator1/1 -> Switch/2
  Delay31/1 -> pixelBusGenerator/1(validIn)
  Logical Operator2/1 -> HDL Counter/1
  Bus Selector/1 -> Delay1/1  "<vStart>"
  Bus Selector1/1 -> Delay6/1  "<vStart>"
  leftBus/1 -> Bus Selector/1
  rightBus/1 -> Bus Selector1/1
  Delay/1 -> Logical Operator/1
  Delay3/1 -> Logical Operator/2, enabledTappedDelay/Enable
  Delay4/1 -> Int2Bin/1(intIn)
  Delay5/1 -> enabledTappedDelay/1(pixelIn)
  Delay2/1 -> Delay3/1
  Delay6/1 -> Logical Operator2/2
  Delay1/1 -> Logical Operator2/1
  Delay7/1 -> Delay/1

== system SGBMDisparity/SGBMHDLAlgorithm/SGBMHDLAlgorithmWorker/MatchingCost/HammDistRL ==
  leftIn : Inport
  leftBus : Inport  Port=2
  rightIn : Inport  Port=3
  rightBus : Inport  Port=4
  CC9 : simulink/Logic and Bit Operations/Compare To Constant  relop=<  const=imgColSize-1  OutDataTypeStr=boolean
  Compare To Constant8 : simulink/Logic and Bit Operations/Compare To Constant  relop=>=  const=disparityLevels-1  OutDataTypeStr=boolean
  Constant4 : Constant  Value=0  OutDataTypeStr=boolean  SampleTime=-1
  Constant5 : Constant  OutDataTypeStr=boolean  SampleTime=-1
  Delay31 : Delay  DelayLength=5
  Delay64 : Delay  DelayLength=disparityLevels - 1  ShowEnablePort=on
      settings: InputPortMap=u0,e6
  HDL Counter16 : hdlsllib/Sources/HDL Counter  CountType=Count limited  CountInit=0  CountStep=1  CountMax=imgColSize-1  CountFromType=Initial value  CountFrom=0  CountResetPort=on  CountLoadPort=off  CountEnbPort=on  CountDirPort=off  CountHitOutputPort=off  CountDataType=Unsigned  CountWordLen=ceil(log2(imgColSize))  CountFracLen=0  CountSampTime=1
  Int2Bin : Subsystem
  Logical Operator1 : Logic  AllPortsSameDT=off  OutDataTypeStr=boolean
  Logical Operator2 : Logic  AllPortsSameDT=off  OutDataTypeStr=boolean
  Logical Operator3 : Logic  Inputs=3  AllPortsSameDT=off  OutDataTypeStr=boolean
  Switch4 : Switch  Criteria=u2 ~= 0
  enabledTappedDelay : Subsystem
  hammDispForEach : Subsystem  TreatAsAtomicUnit=on
  inverseRowLeft : Subsystem
  inverseRowLeft1 : Subsystem
  pixelBusGenerator : Subsystem  mask{hEnd=r, vEnd=s}
      mask prompts: hEnd "hEnd Count"; vEnd "vEnd Count"
      mask DialogControl DescGroupVar Prompt: Counter Values
  hammDist : Outport  VectorParamsAs1DForOutWhenUnconnected=off
  busOut : Outport  Port=2  VectorParamsAs1DForOutWhenUnconnected=off
  wires:
  Logical Operator2/1 -> Logical Operator3/3, HDL Counter16/2
  Constant4/1 -> Switch4/3
  Constant5/1 -> Switch4/1
  Switch4/1 -> Delay31/1
  Delay31/1 -> pixelBusGenerator/1(validIn)
  CC9/1 -> Logical Operator3/2
  Compare To Constant8/1 -> Logical Operator3/1
  Logical Operator3/1 -> Switch4/2
  Delay64/1 -> Int2Bin/1(intIn)
  pixelBusGenerator/1(busOut) -> busOut/1
  hammDispForEach/1(hammDist) -> hammDist/1
  rightIn/1 -> inverseRowLeft1/1(rightIn)
  rightBus/1 -> inverseRowLeft1/2(rightBus)
  inverseRowLeft1/1(rightValid) -> enabledTappedDelay/Enable, Logical Operator2/2
  leftIn/1 -> inverseRowLeft/1(leftIn)
  leftBus/1 -> inverseRowLeft/2(leftBus)
  inverseRowLeft/1(leftValid) -> Delay64/2, Logical Operator2/1
  inverseRowLeft/2(leftOut) -> Delay64/1
  Int2Bin/1(binOut) -> hammDispForEach/1(leftCSCTIn)
  enabledTappedDelay/1(pixelOut) -> hammDispForEach/2(rightCSCTIn)
  inverseRowLeft1/2(rightOut) -> enabledTappedDelay/1(pixelIn)
  HDL Counter16/1 -> CC9/1, Compare To Constant8/1
  Logical Operator1/1 -> HDL Counter16/1
  inverseRowLeft1/3(rightvStart) -> Logical Operator1/2
  inverseRowLeft/3(leftvStart) -> Logical Operator1/1

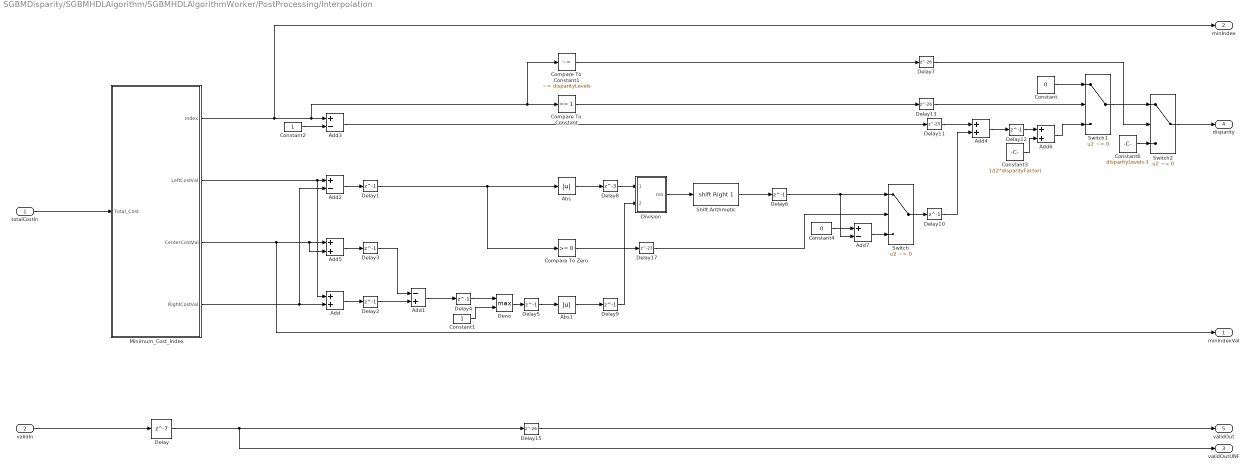
== system SGBMDisparity/SGBMHDLAlgorithm/SGBMHDLAlgorithmWorker/PostProcessing/Interpolation ==
  totalCostIn : Inport
  validIn : Inport  Port=2
  Abs : Abs  OutDataTypeStr=fixdt(0,13,0)  RndMeth=Nearest  SaturateOnIntegerOverflow=on
  Abs1 : Abs  OutDataTypeStr=fixdt(0,13,0)  RndMeth=Nearest  SaturateOnIntegerOverflow=on
  Add{,4..6} (4 alike) : Sum
  Add1 : Sum  Inputs=-+  OutDataTypeStr=fixdt(1,13,0)
  Add2 : Sum  Inputs=+-
  Add3 : Sum  Inputs=+-  OutDataTypeStr=uint8
  Add7 : Sum  Inputs=+-
  Compare To Constant : simulink/Logic and Bit Operations/Compare To Constant  relop===  const=1  OutDataTypeStr=boolean
  Compare To Constant1 : simulink/Logic and Bit Operations/Compare To Constant  relop=~=  const=disparityLevels  OutDataTypeStr=boolean
  Compare To Zero : simulink/Logic and Bit Operations/Compare To Zero  relop=>=  OutDataTypeStr=boolean
  Constant : Constant  Value=0  OutDataTypeStr=fixdt(1,19,4)  SampleTime=-1
  Constant1 : Constant  OutDataTypeStr=fixdt(1,13,0)  SampleTime=-1
  Constant2 : Constant  OutDataTypeStr=fixdt(0,1,0)  SampleTime=-1
  Constant3 : Constant  Value=1/(2*disparityFactor)  OutDataTypeStr=fixdt(1,17,8)  SampleTime=-1
  Constant4 : Constant  Value=0  OutDataTypeStr=fixdt(0,1,0)  SampleTime=-1
  Constant6 : Constant  Value=disparityLevels-1  OutDataTypeStr=fixdt(1,19,4)  SampleTime=-1
  Delay : Delay  DelayLength=7
  Delay{1..6,9..10,12} (9 alike) : Delay  DelayLength=1
  Delay11 : Delay  DelayLength=25
  Delay13 : Delay  DelayLength=26
  Delay15 : Delay  DelayLength=26
  Delay17 : Delay  DelayLength=23
  Delay7 : Delay  DelayLength=26
  Delay8 : Delay  DelayLength=3
  Deno : MinMax  Function=max  Inputs=2  RndMeth=Simplest  SaturateOnIntegerOverflow=on
  Division : Subsystem
  Minimum_Cost_Index : Subsystem
  Shift Arithmetic : ArithShift  BitShiftNumber=1  BitShiftDirection=Right
  Switch : Switch  Criteria=u2 ~= 0
  Switch1 : Switch  Criteria=u2 ~= 0
  Switch2 : Switch  Criteria=u2 ~= 0
  minIndexVal : Outport  VectorParamsAs1DForOutWhenUnconnected=off
  minIndex : Outport  Port=2  VectorParamsAs1DForOutWhenUnconnected=off
  validOutUNF : Outport  Port=3  VectorParamsAs1DForOutWhenUnconnected=off
  disparity : Outport  Port=4  VectorParamsAs1DForOutWhenUnconnected=off
  validOut : Outport  Port=5  VectorParamsAs1DForOutWhenUnconnected=off
  wires:
  validIn/1 -> Delay/1
  totalCostIn/1 -> Minimum_Cost_Index/1(Total_Cost)
  Minimum_Cost_Index/2(LeftCostVal) -> Add/1, Add2/1
  Minimum_Cost_Index/4(RightCostVal) -> Add/2, Add2/2
  Minimum_Cost_Index/1(Index) -> Compare To Constant/1, Compare To Constant1/1, Add3/1, minIndex/1
  Minimum_Cost_Index/3(CenterCostVal) -> Add5/2, Add5/1, minIndexVal/1
  Add/1 -> Delay2/1
  Add5/1 -> Delay3/1
  Add1/1 -> Delay4/1
  Delay4/1 -> Deno/1
  Constant1/1 -> Deno/2
  Deno/1 -> Delay5/1
  Add2/1 -> Delay1/1
  Delay2/1 -> Add1/2
  Delay3/1 -> Add1/1
  Delay1/1 -> Abs/1, Compare To Zero/1
  Abs/1 -> Delay8/1
  Delay8/1 -> Division/1(Dividend)
  Delay5/1 -> Abs1/1
  Abs1/1 -> Delay9/1
  Delay9/1 -> Division/2(Divisor)
  Constant2/1 -> Add3/2
  Add3/1 -> Delay11/1
  Delay11/1 -> Add4/1
  Delay10/1 -> Add4/2
  Add4/1 -> Delay12/1
  Delay12/1 -> Add6/1
  Constant3/1 -> Add6/2
  Switch/1 -> Delay10/1
  Compare To Zero/1 -> Delay17/1
  Add7/1 -> Switch/3
  Constant4/1 -> Add7/1
  Division/1(res) -> Shift Arithmetic/1
  Delay15/1 -> validOut/1
  Shift Arithmetic/1 -> Delay6/1
  Delay6/1 -> Switch/1, Add7/2
  Delay17/1 -> Switch/2
  Delay/1 -> Delay15/1, validOutUNF/1
  Add6/1 -> Switch1/3
  Switch1/1 -> Switch2/1
  Compare To Constant/1 -> Delay13/1
  Compare To Constant1/1 -> Delay7/1
  Constant/1 -> Switch1/1
  Constant6/1 -> Switch2/3
  Switch2/1 -> disparity/1
  Delay7/1 -> Switch2/2
  Delay13/1 -> Switch1/2

== system SGBMDisparity/SGBMHDLAlgorithm/SGBMHDLAlgorithmWorker/PostProcessing/UniquenessFcn ==
  totalCostIn : Inport
  minIndexVal : Inport  Port=2
  minIndex : Inport  Port=3
  validIn : Inport  Port=4
  Add : Sum  Inputs=+-
  Constant : Constant  Value=uniquenessRatio  OutDataTypeStr=uint8  SampleTime=-1
  Constant2 : Constant  Value=100  OutDataTypeStr=uint8  SampleTime=-1
  Constant3 : Constant  Value=100  OutDataTypeStr=uint8  SampleTime=-1
  Delay{,1..2,4,131,134..135} (7 alike) : Delay  DelayLength=1
  Delay3 : Delay  DelayLength=5
  For Each Subsystem : Subsystem  TreatAsAtomicUnit=on
  For Each Subsystem1 : Subsystem  TreatAsAtomicUnit=on
  Index : Constant  Value=[1:disparityLevels]  OutDataTypeStr=uint8  SampleTime=-1
  Logical Operator : Logic  AllPortsSameDT=off  OutDataTypeStr=boolean
  Logical Operator1 : Logic  Operator=OR  Inputs=1  AllPortsSameDT=off  OutDataTypeStr=boolean
  Product1 : Product  RndMeth=Simplest
  UNF : Outport  VectorParamsAs1DForOutWhenUnconnected=off
  validOut : Outport  Port=2  VectorParamsAs1DForOutWhenUnconnected=off
  wires:
  validIn/1 -> Delay3/1
  Delay3/1 -> validOut/1
  Logical Operator/1 -> Delay2/1
  Constant3/1 -> Product1/2
  Product1/1 -> Delay131/1
  Delay135/1 -> Product1/1
  Delay131/1 -> For Each Subsystem/3(min_index_val)
  Add/1 -> For Each Subsystem/2(total_cost1)
  Constant/1 -> Add/2
  Constant2/1 -> Add/1
  Delay134/1 -> For Each Subsystem/1(total_cost)
  minIndexVal/1 -> Delay135/1
  totalCostIn/1 -> Delay134/1
  Index/1 -> For Each Subsystem1/2(Index)
  For Each Subsystem/1(Out1) -> Delay/1
  For Each Subsystem1/1(Out1) -> Delay1/1
  Delay/1 -> Logical Operator/1
  Delay1/1 -> Logical Operator/2
  minIndex/1 -> For Each Subsystem1/1(min_Index)
  Logical Operator1/1 -> Delay4/1
  Delay2/1 -> Logical Operator1/1
  Delay4/1 -> UNF/1

== system SGBMDisparity/SGBMHDLAlgorithm/SGBMHDLAlgorithmWorker/PostProcessing/pixelBusGenerator ==
  validIn : Inport
  Horizontal : hdlsllib/Sources/HDL Counter  CountType=Count limited  CountInit=0  CountStep=1  CountMax=hEnd  CountFromType=Initial value  CountFrom=0  CountResetPort=off  CountLoadPort=off  CountEnbPort=on  CountDirPort=off  CountHitOutputPort=off  CountDataType=Unsigned  CountWordLen=ceil(log2(hEnd))  CountFracLen=0  CountSampTime=1
  Logical Operator{3..6} (4 alike) : Logic  AllPortsSameDT=off  OutDataTypeStr=boolean
  Pixel Control Bus Creator : visionhdlutilities/Pixel Control Bus Creator
      settings: SourceProductBaseCode=VT
  Vertical : hdlsllib/Sources/HDL Counter  CountType=Count limited  CountInit=0  CountStep=1  CountMax=vEnd  CountFromType=Initial value  CountFrom=0  CountResetPort=off  CountLoadPort=off  CountEnbPort=on  CountDirPort=off  CountHitOutputPort=off  CountDataType=Unsigned  CountWordLen=ceil(log2(vEnd))  CountFracLen=0  CountSampTime=1
  hEnd : simulink/Logic and Bit Operations/Compare To Constant  relop===  const=hEnd  OutDataTypeStr=boolean
  hStart : simulink/Logic and Bit Operations/Compare To Constant  relop===  const=0  OutDataTypeStr=boolean
  vEnd : simulink/Logic and Bit Operations/Compare To Constant  relop===  const=vEnd  OutDataTypeStr=boolean
  vStart : simulink/Logic and Bit Operations/Compare To Constant  relop===  const=0  OutDataTypeStr=boolean
  busOut : Outport  VectorParamsAs1DForOutWhenUnconnected=off
  wires:
  validIn/1 -> Pixel Control Bus Creator/5, Vertical/1, Logical Operator4/1, Logical Operator5/1, Logical Operator6/1, Logical Operator3/1, Horizontal/1
  Horizontal/1 -> hEnd/1, hStart/1
  hEnd/1 -> Logical Operator4/2
  Vertical/1 -> vStart/1, vEnd/1
  vStart/1 -> Logical Operator5/2
  vEnd/1 -> Logical Operator6/2
  Logical Operator5/1 -> Pixel Control Bus Creator/3
  Logical Operator3/1 -> Pixel Control Bus Creator/1
  Logical Operator4/1 -> Pixel Control Bus Creator/2
  hStart/1 -> Logical Operator3/2
  Logical Operator6/1 -> Pixel Control Bus Creator/4
  Pixel Control Bus Creator/1 -> busOut/1

== system SGBMDisparity/SGBMHDLAlgorithm/SGBMHDLAlgorithmWorker/DirectionalCost/LeftToRight/lrSubsystem ==
  enable : Inport
  matchCostIn : Inport  Port=2
  Enable : EnablePort
  Delay : Delay  DelayLength=1
  For Each Subsystem : Subsystem  TreatAsAtomicUnit=on
  MinMax1 : MinMax  ZeroCross=off
  Signal Specification : SignalSpecification  Dimensions=disparityLevels
  Switch32 : Switch  Criteria=u2 ~= 0
  d+1 : Subsystem
  d-1 : Subsystem
  minCostPath : Subsystem  TreatAsAtomicUnit=on
  lrCost : Outport  InitialOutput=0  VectorParamsAs1DForOutWhenUnconnected=off
  wires:
  Delay/1 -> MinMax1/1, minCostPath/2(prevCost_d), d+1/1(prevCost_d), d-1/1(prevCost_d)
  MinMax1/1 -> minCostPath/5(minPrevCost)
  d+1/1(prevCost_d+1) -> minCostPath/4(prevCost_d+1)
  minCostPath/1(currCost) -> Switch32/1, Signal Specification/1, lrCost/1
  Switch32/1 -> Delay/1
  d-1/1(prevCost_d-1) -> minCostPath/3(prevCost_d-1)
  For Each Subsystem/1(Out1) -> Switch32/3
  Signal Specification/1 -> For Each Subsystem/1(In1)
  matchCostIn/1 -> minCostPath/1(matchingCost)
  enable/1 -> Switch32/2
